simulink model "bpsk6"  (R2020b)
settings: Solver=VariableStepAuto  StartTime=0.0  StopTime=500  RelTol=1e-3
undefined symbols (not defined in the file): j
libraries: dsp_blocks x7
settings Model: Creator=hp  LastModifiedBy=hp

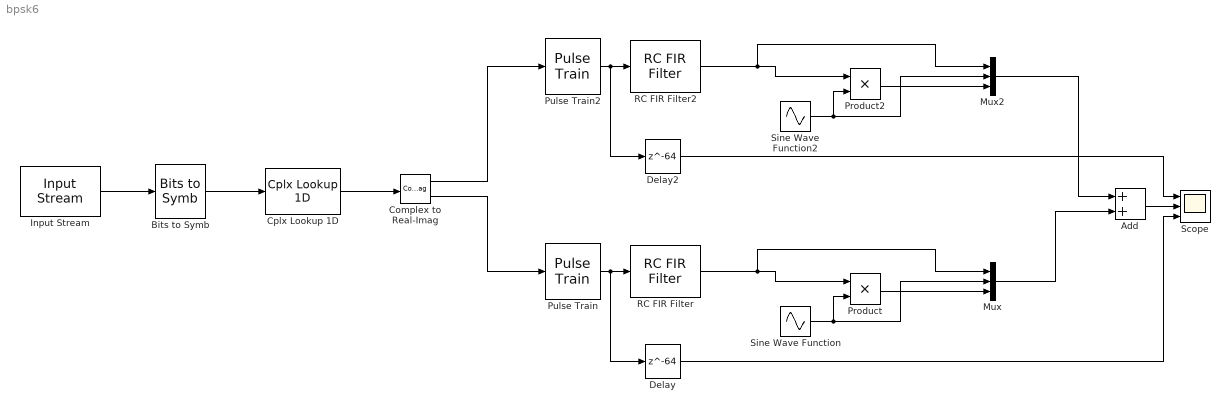
== system bpsk6 ==
  Add : Sum
  Bits to Symb : dsp_blocks/Conversions/Bits to Symb
  Complex to Real-Imag : ComplexToRealImag
  Cplx Lookup 1D : dsp_blocks/Conversions/Cplx Lookup 1D  table=[1 j -1 -j]
  Delay : Delay  DelayLength=64
  Delay2 : Delay  DelayLength=64
  Input Stream : dsp_blocks/Sources//Sinks/Input Stream  period=50  width=2  fname=rand.mat
  Mux : Mux  Inputs=3
  Mux2 : Mux  Inputs=3
  Product : Product
  Product2 : Product
  Pulse Train : dsp_blocks/Conversions/Pulse Train  period=50
  Pulse Train2 : dsp_blocks/Conversions/Pulse Train  period=50
  RC FIR Filter : dsp_blocks/Filters/RC FIR Filter  period=50  beta=0.5  root=off  filt_len=128  win_type=on
  RC FIR Filter2 : dsp_blocks/Filters/RC FIR Filter  period=50  beta=0.5  root=off  filt_len=128  win_type=on
  Scope : Scope  NumInputPorts=3
  Sine Wave Function : Sin  Frequency=2*pi*0.1  Phase=pi  SampleTime=0
  Sine Wave Function2 : Sin  Frequency=2*pi*0.1  Phase=pi/2  SampleTime=0
  wires:
  Input Stream/1 -> Bits to Symb/1
  Bits to Symb/1 -> Cplx Lookup 1D/1
  Pulse Train/1 -> Delay/1, RC FIR Filter/1
  Delay/1 -> Scope/3
  Mux/1 -> Add/2
  Product/1 -> Mux/3
  Sine Wave Function/1 -> Product/2, Mux/2
  RC FIR Filter/1 -> Mux/1, Product/1
  Pulse Train2/1 -> Delay2/1, RC FIR Filter2/1
  Delay2/1 -> Scope/1
  Complex to Real-Imag/1 -> Pulse Train2/1
  RC FIR Filter2/1 -> Mux2/1, Product2/1
  Sine Wave Function2/1 -> Product2/2, Mux2/2
  Product2/1 -> Mux2/3
  Mux2/1 -> Add/1
  Complex to Real-Imag/2 -> Pulse Train/1
  Add/1 -> Scope/2
  Cplx Lookup 1D/1 -> Complex to Real-Imag/1
